simulink model "fin_simu_continuous"  (R2022a)
settings: Solver=ode45  StartTime=0.0  StopTime=time  RelTol=1e-8  AbsTol=1e-10
values from neighbouring files (symbols this model uses):
  b0 = b0(~all(isnan(b0),2), :)    [getNN_simu.m]
  b1 = b1(~all(isnan(b1),2), :)    [getNN_simu.m]
  b2 = b2(1)    [getNN_simu.m]
  gamma = 10000    [code_simu_continuous.m]    (also in code_simu_continuous_1.m)
  mu_x = mu_x(:)    [getNN_simu.m]
  mu_y = Ty.mean(1)    [getNN_simu.m]
  omega = 3.14159265*0.1    (= 0.314159265)    [code_simu_continuous.m]    (also in code_simu_continuous_1.m)
  ran_max = 20    [code_simu_continuous.m]    (also in code_simu_continuous_1.m)
  ran_min = 5    [code_simu_continuous.m]    (also in code_simu_continuous_1.m)
  rho = -2    [code_simu_continuous.m]    (also in code_simu_continuous_1.m)
  seed = 1    [code_simu_continuous.m]    (also in code_simu_continuous_1.m)
  sig_x = sig_x(:)    [getNN_simu.m]
  sig_y = Ty.std(1)    [getNN_simu.m]
  sigma = 0.1    [code_simu_continuous.m]    (also in code_simu_continuous_1.m)
  Td = 0.005    [code_simu_continuous.m]    (also in code_simu_continuous_1.m)
  w0 = w0(~all(isnan(w0),2), ~all(isnan(w0),1))    [getNN_simu.m]
  w1 = w1(~all(isnan(w1),2), ~all(isnan(w1),1))    [getNN_simu.m]
  w2 = w2(~all(isnan(w2),2), :)    [getNN_simu.m]
  wav = 1.5    [code_simu_continuous.m]    (also in code_simu_continuous_1.m)
undefined symbols (not defined in the file or in its folder): A0, AA_s, AT, B0, BB_s, BT, C0, CC_s, CT, D0, DD_s, DT
libraries: simulink x1
settings Model: Creator=IDS_PC  LastModifiedBy=IDS_PC
settings SolverCC: SolverResetMethod=Robust
settings DebuggingCC: AlgebraicLoopMsg=none

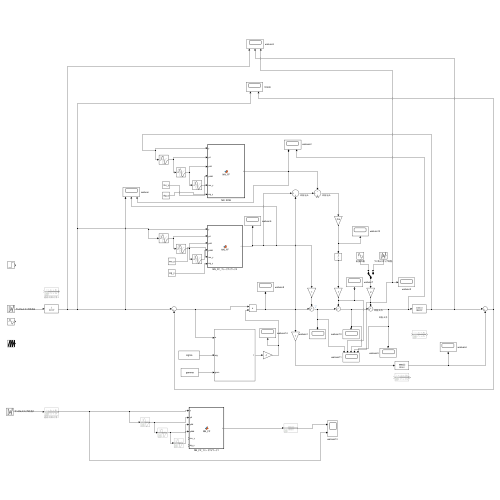
[thumbnail: Simulink's stored preview of the top-level diagram]
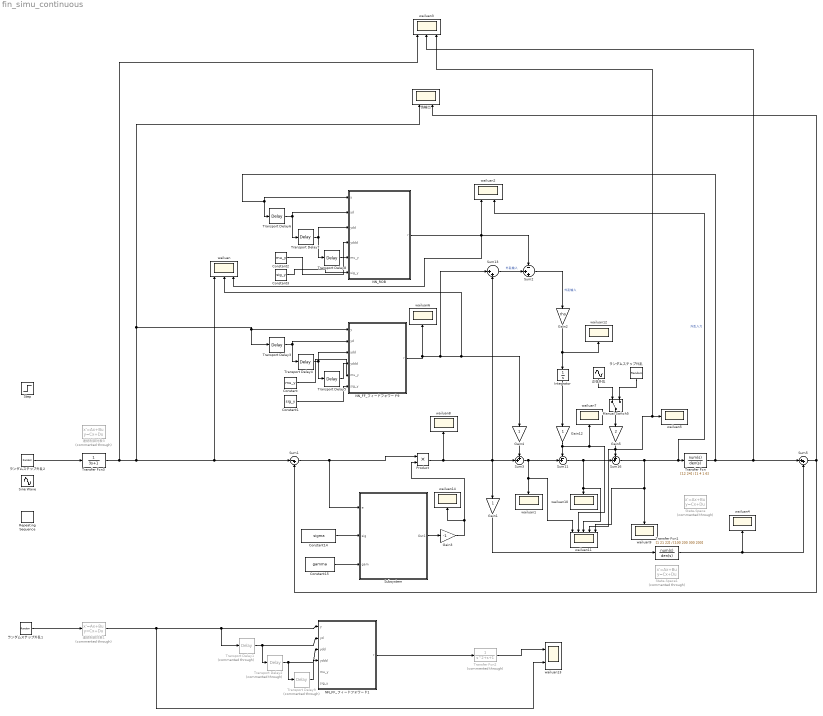
== system fin_simu_continuous ==
  " 正弦外乱" : Sin  Amplitude=wav  Frequency=omega  Phase=1  SampleTime=0
  Constant : Constant  Value=mu_y
  Constant1 : Constant  Value=sig_y
  Constant14 : Constant  Value=sigma  SampleTime=0
  Constant15 : Constant  Value=gamma  SampleTime=0
  Constant2 : Constant  Value=mu_y
  Constant3 : Constant  Value=sig_y
  Gain1 : Gain
  Gain12 : Gain
  Gain2 : Gain  Gain=rho
  Gain3 : Gain  Gain=-1
  Gain4 : Gain
  Gain5 : Gain  Gain=2
  Integrator : Integrator
  Manual Switch5 : ManualSwitch
  NN_FF_フィードフォワード1 : MATLAB Function  TreatAsAtomicUnit=on
  NN_FF_フィードフォワード9 : MATLAB Function  TreatAsAtomicUnit=on
  NN_ROB : MATLAB Function  TreatAsAtomicUnit=on
  Product : Product
  Repeating Sequence : simulink/Sources/Repeating Sequence  rep_seq_t=[0 2]  rep_seq_y=[0 2]
  Sine Wave : Sin  SampleTime=0
  State-Space : StateSpace  Commented=through  A=AT  B=BT  C=CT  D=DT  InitialCondition=0
  State-Space1 : StateSpace  Commented=through  A=AA_s  B=BB_s  C=CC_s  D=DD_s  InitialCondition=0
  Step : Step  SampleTime=0
  Subsystem : Subsystem
  Sum1 : Sum  Inputs=|-+
  Sum11 : Sum  Inputs=-+|
  Sum13 : Sum  Inputs=|++
  Sum16 : Sum  Inputs=++|
  Sum2 : Sum  Inputs=-++
  Sum3 : Sum  Inputs=++|
  Sum5 : Sum  Inputs=|++
  Transfer Fcn : TransferFcn  Numerator=[12 24]  Denominator=[1 4 1 6]
  Transfer Fcn1 : TransferFcn  Numerator=[1 21 22]  Denominator=[100 200 300 200]
  Transfer Fcn2 : TransferFcn  Commented=through  Denominator=[1 1 1]
  Transfer Fcn3 : TransferFcn  Denominator=[3 1]
  Transport Delay1 : TransportDelay  Commented=through  DelayTime=Td
  Transport Delay2 : TransportDelay  Commented=through  DelayTime=Td
  Transport Delay{3..8} (6 alike) : TransportDelay  DelayTime=Td
  Transport Delay9 : TransportDelay  Commented=through  DelayTime=Td
  wailuan : Scope  NumInputPorts=3
  wailuan{1,4..10,12,14} (10 alike) : Scope
  wailuan11 : Scope  NumInputPorts=5
  wailuan13 : Scope  NumInputPorts=2
  wailuan2 : Scope  NumInputPorts=2
  wailuan3 : Scope  NumInputPorts=3
  ランダムステップ外乱 : UniformRandomNumber  Minimum=-wav  Maximum=wav  Seed=seed  SampleTime=16
  ランダムステップ外乱1 : UniformRandomNumber  Minimum=ran_min  Maximum=ran_max  Seed=seed  SampleTime=32
  ランダムステップ外乱2 : UniformRandomNumber  Minimum=ran_min  Maximum=ran_max  Seed=seed  SampleTime=32
  伪输出 : Scope  NumInputPorts=2
  連続制御対象1 : StateSpace  Commented=through  A=A0  B=B0  C=C0  D=D0  InitialCondition=0
  連続制御対象3 : StateSpace  Commented=through  A=A0  B=B0  C=C0  D=D0  InitialCondition=0
  wires:
  Sum16/1 -> wailuan2/2, Transfer Fcn/1, wailuan11/5, wailuan9/1  "外乱入力"
  Gain5/1 -> wailuan11/4, wailuan3/3, wailuan5/1, Sum16/1
  Manual Switch5/1 -> Gain5/1
  ランダムステップ外乱/1 -> Manual Switch5/2
  " 正弦外乱"/1 -> Manual Switch5/1
  Sum11/1 -> Sum16/2, wailuan11/3, wailuan10/1
  Gain12/1 -> Sum11/1, wailuan11/2, wailuan7/1
  Product/1 -> Gain1/1, Sum3/2, Sum13/2, wailuan8/1
  Transfer Fcn/1 -> wailuan3/2, Sum5/1, Transport Delay6/1, NN_ROB/1(y)
  Transfer Fcn3/1 -> wailuan3/1, Sum1/1, wailuan/1, 伪输出/1, Transport Delay3/1, NN_FF_フィードフォワード9/1(y)
  NN_FF_フィードフォワード9/1(r) -> wailuan6/1, Sum13/1, wailuan/2, Gain4/1
  NN_ROB/1(r) -> wailuan2/1, Sum2/1, wailuan/3
  Sum13/1 -> Sum2/2  "外乱输入"
  Gain2/1 -> wailuan12/1, Integrator/1
  Sum2/1 -> Gain2/1  "外乱输入"
  Integrator/1 -> Gain12/1
  Transport Delay5/1 -> NN_FF_フィードフォワード9/4(yddd)
  Transport Delay4/1 -> Transport Delay5/1, NN_FF_フィードフォワード9/3(ydd)
  Transport Delay3/1 -> Transport Delay4/1, NN_FF_フィードフォワード9/2(yd)
  Transport Delay8/1 -> NN_ROB/4(yddd)
  Transport Delay6/1 -> Transport Delay7/1, NN_ROB/2(yd)
  Transport Delay7/1 -> Transport Delay8/1, NN_ROB/3(ydd)
  Gain1/1 -> Transfer Fcn1/1
  Transfer Fcn1/1 -> Sum5/2, wailuan4/1
  ランダムステップ外乱2/1 -> Transfer Fcn3/1
  Sum5/1 -> 伪输出/2, Sum1/2
  Sum1/1 -> Product/1, Subsystem/1(e)
  Constant14/1 -> Subsystem/2(sig)
  Constant15/1 -> Subsystem/3(gam)
  Subsystem/1(Out1) -> Gain3/1
  Gain3/1 -> wailuan14/1, Product/2
  Sum3/1 -> Sum11/2, wailuan11/1, wailuan1/1
  ランダムステップ外乱1/1 -> 連続制御対象1/1
  連続制御対象1/1 -> wailuan13/2, Transport Delay1/1, NN_FF_フィードフォワード1/1(y)
  Transport Delay9/1 -> NN_FF_フィードフォワード1/4(yddd)
  Transport Delay2/1 -> Transport Delay9/1, NN_FF_フィードフォワード1/3(ydd)
  Transport Delay1/1 -> Transport Delay2/1, NN_FF_フィードフォワード1/2(yd)
  NN_FF_フィードフォワード1/1(r) -> Transfer Fcn2/1
  Transfer Fcn2/1 -> wailuan13/1
  Constant2/1 -> NN_ROB/5(mu_y)
  Constant3/1 -> NN_ROB/6(sig_y)
  Constant/1 -> NN_FF_フィードフォワード9/5(mu_y)
  Constant1/1 -> NN_FF_フィードフォワード9/6(sig_y)
  Gain4/1 -> Sum3/1

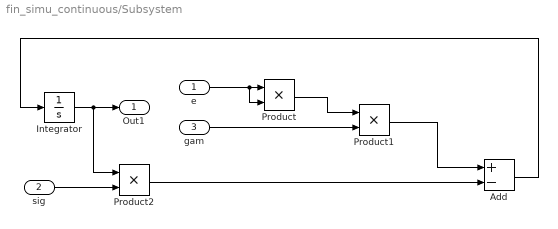
== system fin_simu_continuous/Subsystem ==
  e : Inport
  sig : Inport  Port=2
  gam : Inport  Port=3
  Add : Sum  Inputs=+-
  Integrator : Integrator  UpperSaturationLimit=999999999999999999  LowerSaturationLimit=-9999999999999999
  Product : Product
  Product1 : Product
  Product2 : Product
  Out1 : Outport
  wires:
  e/1 -> Product/2, Product/1
  Product/1 -> Product1/1
  gam/1 -> Product1/2
  Integrator/1 -> Product2/1, Out1/1
  sig/1 -> Product2/2
  Product2/1 -> Add/2
  Product1/1 -> Add/1
  Add/1 -> Integrator/1

== matlab function fin_simu_continuous/NN_ROB ==
  data: y input; yd input; ydd input; yddd input; r output; w0 parameter; b0 parameter; w1 parameter; b1 parameter; w2 parameter; b2 parameter; mu_x parameter; sig_x parameter; mu_y input; sig_y input
function r = NN_FF(y, yd, ydd, yddd, ...
                   w0, b0, w1, b1, w2, b2, ...
                   mu_x, sig_x, mu_y, sig_y)
% y,yd,ydd,yddd: スカラー信号
% w0:[4x64], b0:[64x1], w1:[64x64], b1:[64x1], w2:[64x1], b2:[1x1]
% mu_x,sig_x:[4x1]（入力標準化パラメータ）
% mu_y,sig_y:[1x1]（出力の逆標準化パラメータ）

% 1) 入力標準化
x = [y; yd; ydd; yddd];
x = (x - mu_x) ./ sig_x;

% 2) NN順伝播（Keras: y = W^T x + b）
s1 = (w0.' * x) + b0;  % 64x1
x1 = max(0, s1);

s2 = (w1.' * x1) + b1; % 64x1
x2 = max(0, s2);

s3 = (w2.' * x2) + b2; % 1x1  （標準化空間のr）

% 3) 出力の逆標準化
r = s3 * sig_y + mu_y;

== matlab function fin_simu_continuous/NN_FF_フィードフォワード1 ==
  data: y input; yd input; ydd input; yddd input; r output; w0 parameter; b0 parameter; w1 parameter; b1 parameter; w2 parameter; b2 parameter; mu_x parameter; sig_x parameter; mu_y input; sig_y input
function r = NN_FF(y, yd, ydd, yddd, ...
                   w0, b0, w1, b1, w2, b2, ...
                   mu_x, sig_x, mu_y, sig_y)
% y,yd,ydd,yddd: スカラー信号
% w0:[4x64], b0:[64x1], w1:[64x64], b1:[64x1], w2:[64x1], b2:[1x1]
% mu_x,sig_x:[4x1]（入力標準化パラメータ）
% mu_y,sig_y:[1x1]（出力の逆標準化パラメータ）

% 1) 入力標準化
x = [y; yd; ydd; yddd];
x = (x - mu_x) ./ sig_x;

% 2) NN順伝播（Keras: y = W^T x + b）
s1 = (w0.' * x) + b0;  % 64x1
x1 = max(0, s1);

s2 = (w1.' * x1) + b1; % 64x1
x2 = max(0, s2);

s3 = (w2.' * x2) + b2; % 1x1  （標準化空間のr）

% 3) 出力の逆標準化
r = s3 * sig_y + mu_y;

== matlab function fin_simu_continuous/NN_FF_フィードフォワード9 ==
  data: y input; yd input; ydd input; yddd input; r output; w0 parameter; b0 parameter; w1 parameter; b1 parameter; w2 parameter; b2 parameter; mu_x parameter; sig_x parameter; mu_y input; sig_y input
function r = NN_FF(y, yd, ydd, yddd, ...
                   w0, b0, w1, b1, w2, b2, ...
                   mu_x, sig_x, mu_y, sig_y)
% y,yd,ydd,yddd: スカラー信号
% w0:[4x64], b0:[64x1], w1:[64x64], b1:[64x1], w2:[64x1], b2:[1x1]
% mu_x,sig_x:[4x1]（入力標準化パラメータ）
% mu_y,sig_y:[1x1]（出力の逆標準化パラメータ）

% 1) 入力標準化
x = [y; yd; ydd; yddd];
x = (x - mu_x) ./ sig_x;

% 2) NN順伝播（Keras: y = W^T x + b）
s1 = (w0.' * x) + b0;  % 64x1
x1 = max(0, s1);

s2 = (w1.' * x1) + b1; % 64x1
x2 = max(0, s2);

s3 = (w2.' * x2) + b2; % 1x1  （標準化空間のr）

% 3) 出力の逆標準化
r = s3 * sig_y + mu_y;
